simulink model "sampleModel1551_4"  (R2023a)
settings: Solver=VariableStepAuto  StartTime=0.0  StopTime=10.0  RelTol=1e-3
libraries: hdlsllib x7, simulink x2
settings Model: Creator=user1  LastModifiedBy=user1

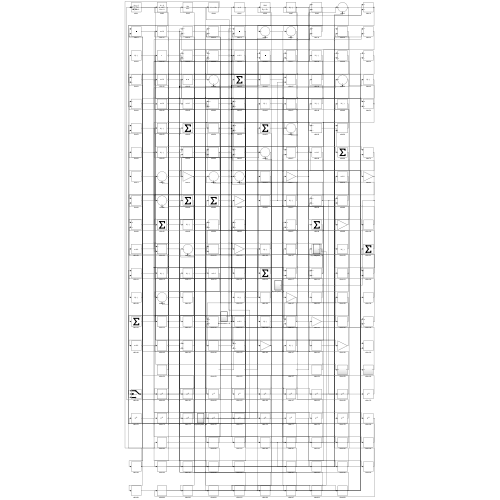
[thumbnail: Simulink's stored preview of the top-level diagram]
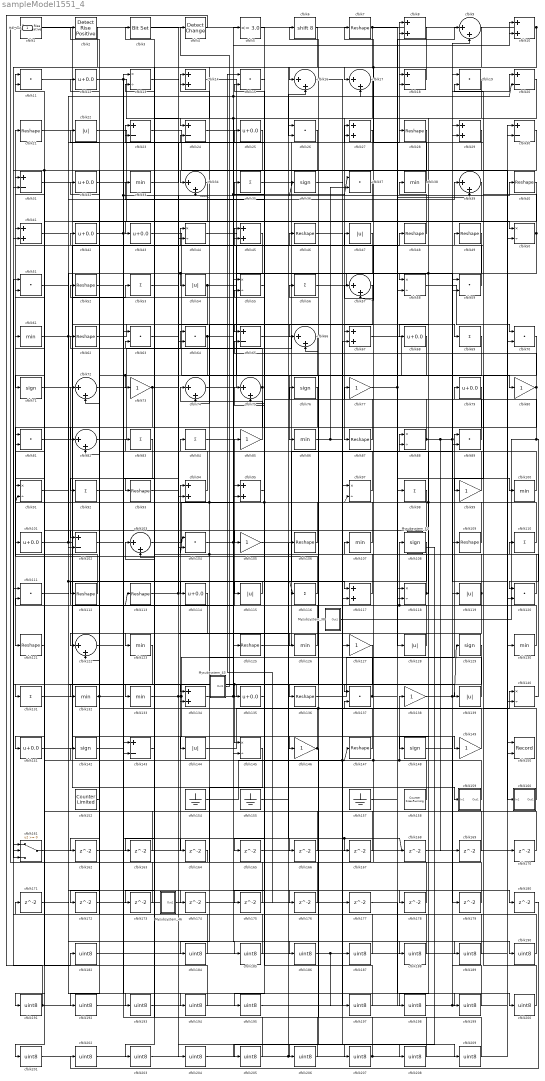
== system sampleModel1551_4 ==
  Mysubsystem_38 : Subsystem  TreatAsAtomicUnit=on  RTWFcnName=Mysubsystem_38
      settings: RTWFcnNameOpts=User specified  RTWFileNameOpts=Use function name
  Mysubsystem_43 : Subsystem  TreatAsAtomicUnit=on  RTWFcnName=Mysubsystem_43
      settings: RTWFcnNameOpts=User specified  RTWFileNameOpts=Use function name
  Mysubsystem_46 : Subsystem  TreatAsAtomicUnit=on  RTWFcnName=Mysubsystem_46
      settings: RTWFcnNameOpts=User specified  RTWFileNameOpts=Use function name
  Mysubsystem_52 : Subsystem  TreatAsAtomicUnit=on  RTWFcnName=Mysubsystem_52
      settings: RTWFcnNameOpts=User specified  RTWFileNameOpts=Use function name
  cfblk1 : hdlsllib/Logic and Bit Operations/Detect Rise Nonnegative  vinit=0  OutDataTypeStr=uint8
  cfblk{8,10,14,27,29,41,45,67,94..95,117,134} (12 alike) : Sum  OutDataTypeStr=uint8
  cfblk{33,38,61,86,100,107,123,126,130,132..133} (11 alike) : MinMax  OutDataTypeStr=uint8
  cfblk{12,25,32,42..43,68,79,101,114,135,141} (11 alike) : Bias  Bias=0.0  SaturateOnIntegerOverflow=off
  cfblk{18,20,23..24,30..31,65,102,143} (9 alike) : Sum  Inputs=+-  OutDataTypeStr=uint8
  cfblk{9,16..17,34,39,57,66,72,74..75,82,103,122} (13 alike) : Sum  Inputs=|++  OutDataTypeStr=uint8
  cfblk{11,15,19,26,37,51,59,63..64,70,81,89,104,111,120,137} (16 alike) : DotProduct  OutDataTypeStr=uint8
  cfblk{73,77,80,85,99,105,127,138,146,149} (10 alike) : Gain  OutDataTypeStr=uint8
  cfblk{7,21,28,40,46,48..49,52,62,87,93,106,109,112..113,121,125,136,147} (19 alike) : Reshape
  cfblk{36,71,76,108,129,142,148} (7 alike) : Signum
  cfblk{35,53,56,69,83..84,92,98,110,116,131} (11 alike) : Sum  Inputs=+  OutDataTypeStr=uint8
  cfblk{22,47,54,115,119,128,139,144} (8 alike) : Abs  OutDataTypeStr=uint8  SaturateOnIntegerOverflow=off
  cfblk{13,44,50,55,58,88,91,97,118,140,145} (11 alike) : Product  Inputs=*/  OutDataTypeStr=uint8  RndMeth=Zero  SaturateOnIntegerOverflow=on
  cfblk150 : Record  FileSettingsInternal="{\"entries\":[{\"content\":{\"excelSettings\":{\"content\":{},\"type\":\"Streamout.ExcelSettings\"}},\"type\":\"Streamout.FileSettingStorage\",\"uuid\":\"\"}],\"packageUris\":[\"http:\\/\\/schema.mathworks.com\\/mf0\\/streamout_blocks\\/R2020a\"],\"version\":\"1.0\"}"  Layout=[1 1]  SignalsInternal="{\"entries\":[{\"content\":{\"signals\":[{\"content\":{\"blockPath\":[],\"dimensions\":[1],\"domain\":\"\",\"lineColor\":\"#a2142f\",\"plots\":[1],\"port\":1,\"signalID\":24250,\"signalName\":\"cfblk67\"},\"type\":\"RecordBlkView.Signal\",\"uuid\":\"\"},{\"content\":{\"blockPath\":[],\"dimensions\":[1],\"domain\":\"\",\"lineColor\":\"#139fff\",\"plots\":[1],\"port\":2,\"signalID\":24253,\"signalName\":\"cfblk186\"},\"type\":\"RecordBlkView.Signal\",\"uuid\":\"\"}]},\"type\":\"RecordBlkView.InputSignals\",\"uuid\":\"\"}],\"packageUris\":[\"http:\\/\\/schema.mathworks.com\\/mf0\\/streamout_blocks\\/R2020a\"],\"version\":\"1.0\"}"  VisualizationBindings="{\"xyplotplugin\":{\"info\":[{\"series\":[{\"bindingParametersList\":[{\"parameter\":\"X-Axis\",\"signalID\":24250,\"signalName\":\"cfblk67\"},{\"parameter\":\"Y-Axis\",\"signalID\":24253,\"signalName\":\"cfblk186\"}],\"seriesID\":65338}],\"subplotID\":1}]}}"  CompatibilityTag=XY  st=-1
  cfblk152 : hdlsllib/Sources/Counter Limited  uplimit=7  tsamp=-1
  cfblk154 : Ground
  cfblk155 : Ground
  cfblk157 : Ground
  cfblk158 : hdlsllib/Sources/Counter Free-Running  NumBits=16  tsamp=-1
  cfblk159 : Subsystem
      settings: LibrarySourceBlock=|
      | hdlsllib/Ports &
      | Subsystems/Subsystem
  cfblk160 : Subsystem
      settings: LibrarySourceBlock=|
      | hdlsllib/Ports &
      | Subsystems/Subsystem
  cfblk161 : Switch  OutDataTypeStr=uint8  SaturateOnIntegerOverflow=off  InputSameDT=off
  cfblk{162..180} (19 alike) : Delay  SampleTime=1
  cfblk{182,184..195,197..209} (26 alike) : DataTypeConversion  OutDataTypeStr=uint8  SaturateOnIntegerOverflow=off  RndMeth=Floor
  cfblk2 : hdlsllib/Logic and Bit Operations/Detect Rise Positive  vinit=0  OutDataTypeStr=uint8
  cfblk3 : simulink/Logic and Bit Operations/Bit Set  iBit=0
      settings: LibrarySourceBlock=|
      | hdlsllib/Logic and Bit
      | Operations/Bit Set
  cfblk4 : simulink/Logic and Bit Operations/Detect Change  vinit=0  OutDataTypeStr=uint8
      settings: LibrarySourceBlock=|
      | hdlsllib/Logic and Bit
      | Operations/Detect
      | Change
  cfblk5 : hdlsllib/Logic and Bit Operations/Compare To Constant  relop=<=  const=3.0  OutDataTypeStr=uint8
  cfblk6 : ArithShift  BitShiftNumber=8
  Hdl_out : Outport  OutDataTypeStr=uint8
  wires:
  cfblk14/1 -> cfblk80/1
  cfblk85/1 -> cfblk74/1
  cfblk62/1 -> cfblk69/1
  cfblk112/1 -> cfblk21/1
  cfblk128/1 -> cfblk108/1, cfblk113/1
  cfblk144/1 -> cfblk140/1
  cfblk75/1 -> cfblk121/1, cfblk2/1
  cfblk141/1 -> cfblk85/1
  cfblk116/1 -> cfblk101/1
  cfblk65/1 -> cfblk117/1
  cfblk136/1 -> cfblk89/1
  cfblk21/1 -> cfblk146/1
  cfblk69/1 -> cfblk105/1
  cfblk81/1 -> cfblk48/1
  cfblk82/1 -> cfblk8/1
  cfblk1/1 -> cfblk66/1
  cfblk161/1 -> cfblk94/1
  cfblk71/1 -> cfblk159/1(In1)
  cfblk34/1 -> cfblk123/1
  cfblk101/1 -> cfblk144/1, cfblk18/2
  cfblk95/1 -> cfblk35/1
  cfblk131/1 -> cfblk53/1
  cfblk159/1(Out1) -> cfblk138/1, cfblk32/1
  cfblk146/1 -> cfblk95/1, cfblk206/1
  cfblk132/1 -> cfblk134/1, cfblk162/1
  cfblk74/1 -> cfblk46/1
  cfblk40/1 -> cfblk91/1
  cfblk130/1 -> cfblk72/1
  cfblk100/1 -> cfblk84/1
  cfblk140/1 -> cfblk110/1
  cfblk66/1 -> cfblk143/2, cfblk73/1
  cfblk24/1 -> cfblk87/1
  cfblk134/1 -> cfblk10/1, cfblk20/2, cfblk137/1
  cfblk43/1 -> cfblk86/1
  cfblk70/1 -> cfblk99/1
  cfblk31/1 -> cfblk43/1
  cfblk64/1 -> cfblk112/1, cfblk190/1
  cfblk35/1 -> cfblk8/2
  cfblk149/1 -> cfblk76/1, cfblk82/2
  cfblk77/1 -> cfblk9/1, cfblk100/1
  cfblk115/1 -> cfblk114/1
  cfblk29/1 -> cfblk34/1
  cfblk117/1 -> cfblk44/1
  cfblk143/1 -> cfblk83/1
  cfblk73/1 -> cfblk131/1, cfblk149/1
  cfblk23/1 -> cfblk160/1(In1)
  cfblk152/1 -> cfblk42/1
  cfblk48/1 -> cfblk38/1
  cfblk80/1 -> cfblk81/1, cfblk65/2
  cfblk138/1 -> cfblk129/1, cfblk10/2
  cfblk129/1 -> cfblk145/1, cfblk161/3
  cfblk45/1 -> cfblk54/1, cfblk102/2
  cfblk27/1 -> cfblk71/1, cfblk41/2
  cfblk125/1 -> cfblk9/2
  cfblk53/1 -> cfblk65/1
  cfblk11/1 -> cfblk50/1
  cfblk59/1 -> cfblk12/1
  cfblk104/1 -> cfblk37/1, cfblk17/2, cfblk125/1
  cfblk56/1 -> cfblk58/1
  cfblk97/1 -> cfblk22/1
  cfblk61/1 -> cfblk117/2, cfblk180/1, cfblk27/2
  cfblk17/1 -> cfblk67/1
  cfblk67/1 -> cfblk150/1
  cfblk33/1 -> cfblk27/1
  cfblk110/1 -> cfblk97/2, cfblk88/2
  cfblk119/1 -> cfblk122/1, cfblk41/1
  cfblk32/1 -> cfblk128/1
  cfblk52/1 -> cfblk94/2
  cfblk89/1 -> cfblk52/1
  cfblk55/1 -> cfblk135/1
  cfblk50/1 -> cfblk68/1, cfblk163/1, cfblk28/1
  cfblk20/1 -> cfblk93/1, cfblk145/2
  cfblk57/1 -> cfblk74/2
  cfblk47/1 -> cfblk92/1
  cfblk94/1 -> cfblk62/1
  cfblk76/1 -> cfblk82/1
  cfblk133/1 -> cfblk95/2, cfblk179/1, cfblk178/1
  cfblk22/1 -> cfblk58/2
  cfblk107/1 -> cfblk23/1
  cfblk139/1 -> cfblk47/1
  cfblk99/1 -> cfblk45/1
  cfblk127/1 -> cfblk141/1
  cfblk103/1 -> cfblk55/1
  cfblk154/1 -> cfblk147/1, cfblk67/2
  cfblk8/1 -> cfblk26/2
  cfblk91/1 -> cfblk25/1
  cfblk37/1 -> cfblk102/1
  cfblk68/1 -> cfblk136/1
  cfblk58/1 -> cfblk70/1
  cfblk113/1 -> cfblk40/1, cfblk126/1
  cfblk7/1 -> cfblk16/1, cfblk50/2
  cfblk158/1 -> cfblk57/1, cfblk51/2
  cfblk42/1 -> cfblk36/1, cfblk18/1, cfblk64/2
  cfblk98/1 -> cfblk191/1
  cfblk142/1 -> cfblk186/1
  cfblk30/1 -> cfblk201/1
  cfblk10/1 -> cfblk57/2, cfblk161/2, Hdl_out/1
  cfblk49/1 -> cfblk148/1
  cfblk157/1 -> cfblk118/1
  cfblk28/1 -> cfblk115/1
  cfblk12/1 -> cfblk44/2, cfblk194/1
  cfblk5/1 -> cfblk75/2
  cfblk83/1 -> cfblk132/1
  cfblk160/1(Out1) -> cfblk79/1
  cfblk118/1 -> cfblk107/1, cfblk88/1
  cfblk39/1 -> cfblk103/2
  cfblk137/1 -> cfblk14/1, cfblk39/2
  cfblk88/1 -> cfblk20/1, cfblk120/2, cfblk169/1, cfblk33/1
  cfblk63/1 -> cfblk207/1
  cfblk72/1 -> cfblk5/1
  cfblk147/1 -> cfblk34/2, cfblk104/1, cfblk6/1
  cfblk123/1 -> cfblk133/1
  cfblk86/1 -> cfblk127/1, cfblk37/2
  cfblk105/1 -> cfblk167/1, cfblk168/1
  cfblk9/1 -> cfblk24/1
  cfblk109/1 -> cfblk24/2
  cfblk51/1 -> cfblk139/1, cfblk116/1
  cfblk44/1 -> cfblk109/1
  cfblk126/1 -> cfblk31/1
  cfblk87/1 -> cfblk23/2
  cfblk120/1 -> cfblk77/1
  cfblk148/1 -> cfblk89/2
  cfblk121/1 -> cfblk11/1
  cfblk2/1 -> cfblk31/2
  cfblk155/1 -> cfblk16/2
  cfblk114/1 -> cfblk122/2
  cfblk18/1 -> cfblk17/1
  cfblk15/1 -> cfblk195/1
  cfblk106/1 -> cfblk91/2, cfblk64/1, cfblk55/2
  cfblk38/1 -> cfblk7/1
  cfblk41/1 -> cfblk39/1
  cfblk54/1 -> cfblk118/2, cfblk104/2
  cfblk162/1 -> cfblk143/1
  cfblk163/1 -> cfblk72/2
  cfblk92/1 -> cfblk164/1
  cfblk164/1 -> cfblk1/1
  cfblk79/1 -> cfblk165/1
  cfblk165/1 -> cfblk29/2
  cfblk93/1 -> cfblk166/1
  cfblk166/1 -> cfblk75/1
  cfblk167/1 -> cfblk14/2
  cfblk168/1 -> cfblk70/2
  cfblk169/1 -> cfblk11/2
  cfblk170/1 -> cfblk66/2
  cfblk108/1 -> cfblk172/1
  cfblk172/1 -> cfblk26/1
  cfblk25/1 -> cfblk173/1
  cfblk173/1 -> cfblk81/2
  cfblk102/1 -> cfblk174/1
  cfblk174/1 -> cfblk97/1
  cfblk135/1 -> cfblk175/1
  cfblk175/1 -> cfblk103/1
  cfblk84/1 -> cfblk176/1
  cfblk176/1 -> cfblk45/2
  cfblk178/1 -> cfblk137/2
  cfblk179/1 -> cfblk134/2
  cfblk4/1 -> cfblk182/1
  cfblk182/1 -> cfblk119/1
  cfblk145/1 -> cfblk184/1
  cfblk184/1 -> cfblk3/1
  cfblk3/1 -> cfblk185/1
  cfblk185/1 -> cfblk161/1
  cfblk186/1 -> cfblk150/2, cfblk197/1
  cfblk46/1 -> cfblk187/1
  cfblk187/1 -> cfblk142/1
  cfblk111/1 -> cfblk188/1
  cfblk188/1 -> cfblk61/1
  cfblk36/1 -> cfblk189/1
  cfblk189/1 -> cfblk111/1
  cfblk190/1 -> cfblk111/2
  cfblk191/1 -> cfblk177/1, cfblk51/1
  cfblk26/1 -> cfblk192/1
  cfblk192/1 -> cfblk98/1
  cfblk171/1 -> cfblk193/1
  cfblk193/1 -> cfblk59/1
  cfblk194/1 -> cfblk171/1
  cfblk195/1 -> cfblk170/1, cfblk59/2
  cfblk197/1 -> cfblk15/2
  cfblk19/1 -> cfblk198/1
  cfblk198/1 -> cfblk29/1
  cfblk122/1 -> cfblk199/1
  cfblk199/1 -> cfblk19/1
  cfblk177/1 -> cfblk200/1
  cfblk200/1 -> cfblk19/2
  cfblk201/1 -> cfblk140/2, cfblk106/1
  cfblk180/1 -> cfblk202/1
  cfblk202/1 -> cfblk30/1
  cfblk6/1 -> cfblk203/1
  cfblk203/1 -> cfblk30/2
  cfblk13/1 -> cfblk204/1
  cfblk205/1 -> cfblk13/1
  cfblk206/1 -> cfblk13/2
  cfblk207/1 -> cfblk56/1, cfblk130/1
  cfblk16/1 -> cfblk208/1
  cfblk208/1 -> cfblk63/1
  cfblk204/1 -> cfblk209/1
  cfblk209/1 -> cfblk63/2
  Mysubsystem_38/1(Out1) -> cfblk49/1, cfblk120/1
  Mysubsystem_43/1(Out1) -> cfblk4/1
  Mysubsystem_46/1(Out1) -> cfblk15/1
  Mysubsystem_52/1(Out1) -> cfblk205/1

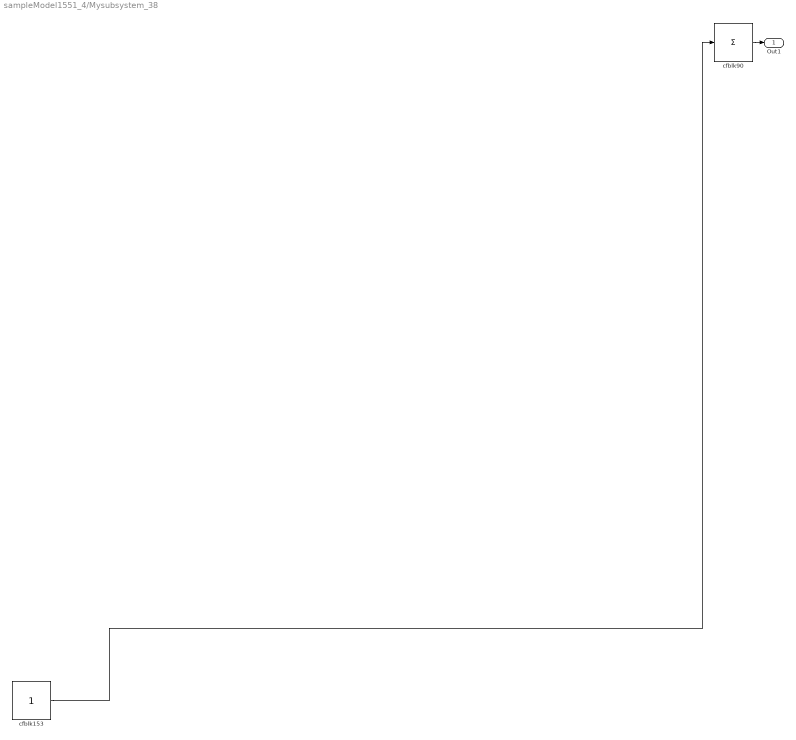
== system sampleModel1551_4/Mysubsystem_38 ==
  cfblk153 : Constant  SampleTime=-1
  cfblk90 : Sum  Inputs=+
  Out1 : Outport
  wires:
  cfblk153/1 -> cfblk90/1
  cfblk90/1 -> Out1/1

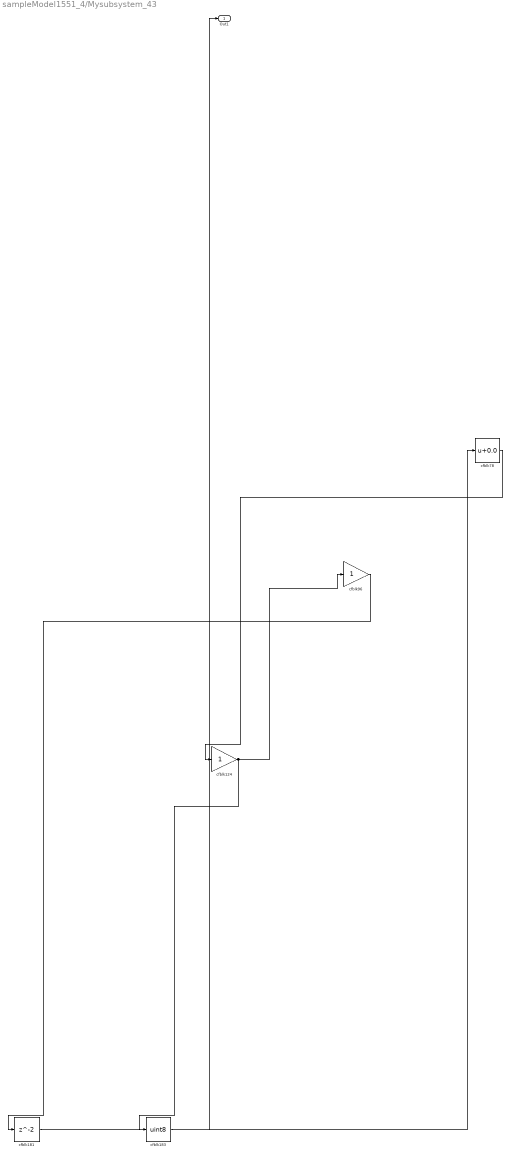
== system sampleModel1551_4/Mysubsystem_43 ==
  cfblk124 : Gain
  cfblk181 : Delay  SampleTime=1
  cfblk183 : DataTypeConversion  OutDataTypeStr=uint8  SaturateOnIntegerOverflow=off  RndMeth=Floor
  cfblk78 : Bias  Bias=0.0  SaturateOnIntegerOverflow=off
  cfblk96 : Gain
  Out1 : Outport
  wires:
  cfblk78/1 -> cfblk124/1
  cfblk181/1 -> cfblk78/1
  cfblk124/1 -> cfblk96/1, cfblk183/1
  cfblk96/1 -> cfblk181/1
  cfblk183/1 -> Out1/1

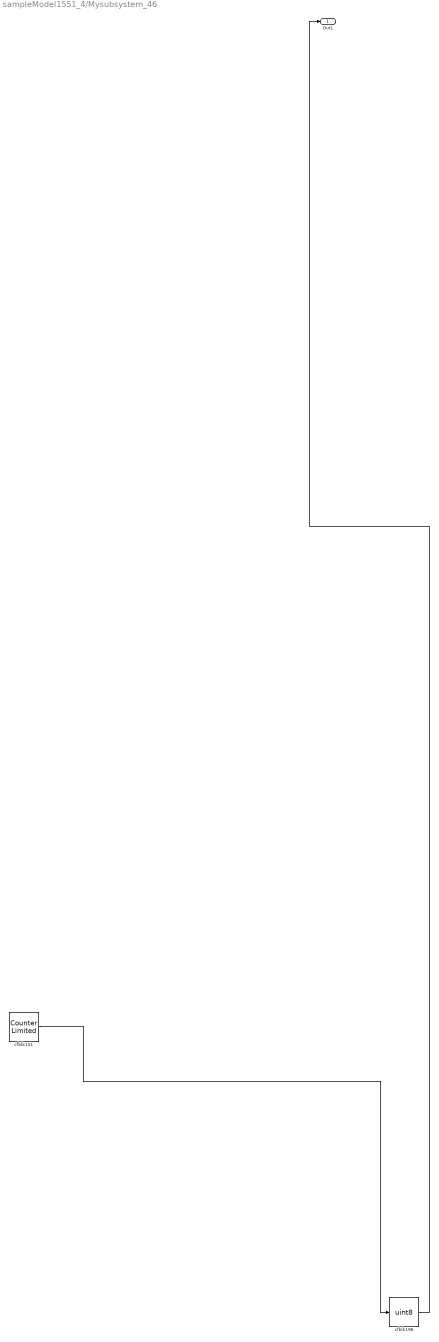
== system sampleModel1551_4/Mysubsystem_46 ==
  cfblk151 : hdlsllib/Sources/Counter Limited  uplimit=7  tsamp=-1
  cfblk196 : DataTypeConversion  OutDataTypeStr=uint8  SaturateOnIntegerOverflow=off  RndMeth=Floor
  Out1 : Outport
  wires:
  cfblk151/1 -> cfblk196/1
  cfblk196/1 -> Out1/1

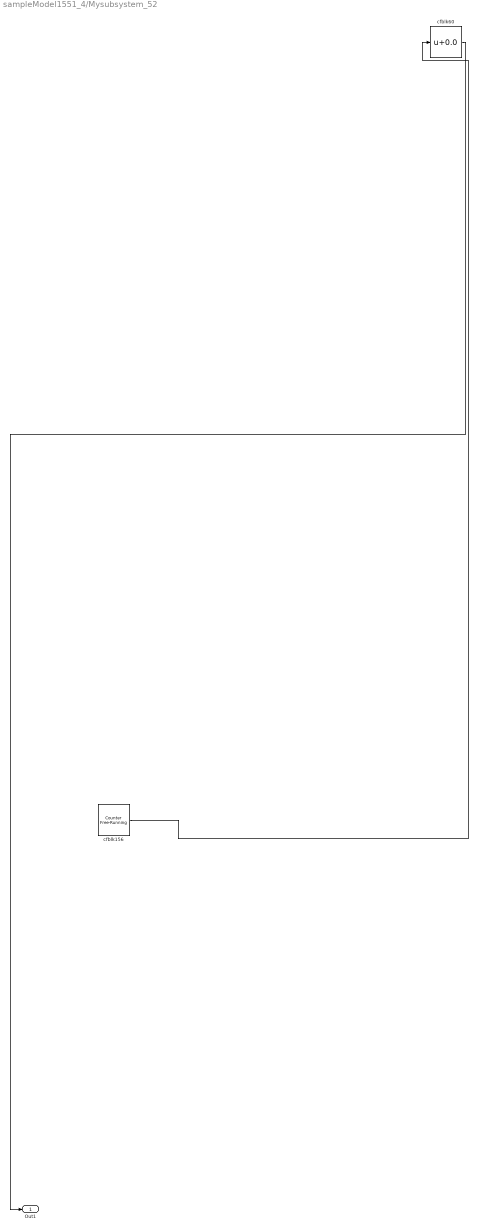
== system sampleModel1551_4/Mysubsystem_52 ==
  cfblk156 : hdlsllib/Sources/Counter Free-Running  NumBits=16  tsamp=-1
  cfblk60 : Bias  Bias=0.0  SaturateOnIntegerOverflow=off
  Out1 : Outport
  wires:
  cfblk60/1 -> Out1/1
  cfblk156/1 -> cfblk60/1

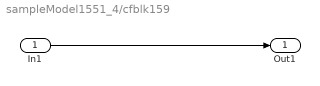
== system sampleModel1551_4/cfblk159 ==
  In1 : Inport
  Out1 : Outport
  wires:
  In1/1 -> Out1/1

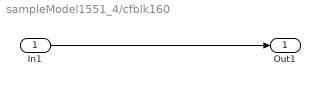
== system sampleModel1551_4/cfblk160 ==
  In1 : Inport
  Out1 : Outport
  wires:
  In1/1 -> Out1/1
